simulink model "bh_model_crank_dynamics"  (R2022b)
settings: Solver=ode15s  StartTime=0.0  StopTime=45  RelTol=1e-4  AbsTol=1e-4  EnableMultiTasking=on
undefined symbols (not defined in the file): IC, params, sigbuilder_block, X, Y, Z
libraries: sm_lib x21, nesl_utility x19, simulink_extras x11, simulink x2
(part 2 of 2)

== system bh_model_crank_dynamics/BRAIN_model/INTEGRATE/Make_BUS/pm_pi ==
  rad_in : Inport
  Trigonometric Function : Trigonometry  Operator=atan2
  Trigonometric Function1 : Trigonometry
  Trigonometric Function2 : Trigonometry  Operator=cos
  rad_out : Outport
  wires:
  rad_in/1 -> Trigonometric Function2/1, Trigonometric Function1/1
  Trigonometric Function2/1 -> Trigonometric Function/2
  Trigonometric Function1/1 -> Trigonometric Function/1
  Trigonometric Function/1 -> rad_out/1

== system bh_model_crank_dynamics/BRAIN_model/INTEGRATE/Make_BUS/pm_pi1 ==
  rad_in : Inport
  Trigonometric Function : Trigonometry  Operator=atan2
  Trigonometric Function1 : Trigonometry
  Trigonometric Function2 : Trigonometry  Operator=cos
  rad_out : Outport
  wires:
  rad_in/1 -> Trigonometric Function2/1, Trigonometric Function1/1
  Trigonometric Function2/1 -> Trigonometric Function/2
  Trigonometric Function1/1 -> Trigonometric Function/1
  Trigonometric Function/1 -> rad_out/1

== matlab function bh_model_crank_dynamics/BRAIN_model/my_EOM1 ==
  data: F_P input; A output; I_A1 input; I_G2 input; L_1 input; L_2 input; b_A input; b_P input; g input; m_1 input; m_2 input; m_P input; tau_A input; theta input; theta_dot input; b output
function [A,b] = my_EOM(F_P,I_A1,I_G2,L_1,L_2,b_A,b_P,g,m_1,m_2,m_P,tau_A,theta,theta_dot)
%#codegen

%    This function was generated by the Symbolic Math Toolbox version 9.2.
%    27-Oct-2022 08:56:04

t2 = cos(theta);
t3 = sin(theta);
t4 = L_1.^2;
t5 = L_1.^3;
t6 = theta_dot.^2;
t10 = 1.0./L_2;
t7 = t2.^2;
t8 = t3.^2;
t9 = L_1.*t3;
t11 = t10.^2;
t12 = L_1.*t2.*t6;
t13 = t6.*t9;
t14 = t9./2.0;
t15 = t4.*t8.*t11;
t16 = -t15;
t17 = t15-1.0;
t18 = t16+1.0;
t19 = 1.0./t17;
t20 = sqrt(t18);
t23 = t3.*t5.*t6.*t7.*t11.*t19;
t21 = 1.0./t20;
t22 = (L_2.*t20)./2.0;
A = reshape([m_1.*t9.*(-1.0./2.0),(L_1.*m_1.*t2)./2.0,I_A1,-m_2.*(t9+(t2.*t3.*t4.*t10.*t21)./2.0),(L_1.*m_2.*t2)./2.0,-I_G2.*L_1.*t2.*t10.*t21,-m_P.*(t9+t2.*t3.*t4.*t10.*t21),0.0,-1.0,0.0,0.0,0.0,0.0,0.0,0.0,0.0,0.0,-1.0,0.0,0.0,0.0,0.0,0.0,0.0,1.0,0.0,-t9,-1.0,0.0,t14,0.0,0.0,0.0,1.0,L_1.*t2,0.0,-1.0,t22,0.0,0.0,0.0,0.0,0.0,1.0,0.0,t14,-1.0,0.0,0.0,0.0,0.0,0.0,1.0,t22,0.0,-1.0,0.0,0.0,0.0,0.0,0.0,0.0,0.0,-1.0],[8,8]);
if nargout > 1
    t24 = t13+t23;
    b = [(m_1.*t12)./2.0;-g.*m_1+(m_1.*t13)./2.0;tau_A-b_A.*theta_dot-(L_1.*g.*m_1.*t2)./2.0;m_2.*(t12-(t9.*t10.*t21.*t24)./2.0+(t4.*t6.*t7.*t10.*t21)./2.0);-g.*m_2+(m_2.*t13)./2.0;-I_G2.*t10.*t21.*t24;F_P+m_P.*(t12-t9.*t10.*t21.*t24+t4.*t6.*t7.*t10.*t21)+b_P.*(t9.*theta_dot+t2.*t3.*t4.*t10.*t21.*theta_dot);-g.*m_P];
end

== matlab function bh_model_crank_dynamics/SIMSCAPE_MODEL/make_R_BUS/Convert_BODY_fixed to WORLD ==
  data: xy_B_vec input size=2; xy_W_vec output size=[2,1]; gamma input size=1
function xy_W_vec = fcn(xy_B_vec, gamma)

    gRb      = [  cos(gamma),  -sin(gamma);
                  sin(gamma),   cos(gamma)   ];
      
    xy_W_vec = gRb * xy_B_vec(:);

end

== matlab function bh_model_crank_dynamics/BRAIN_model/INTEGRATE/CALC_P_pos_and_vel ==
  data: L_1 input; x_P output; L_2 input; theta input; theta_dot input; theta_ddot input; phi input; phi_dot input; v_P output; a_P output; phi_ddot input
function [x_P, v_P, a_P] = fcn(L_1, L_2, theta, theta_dot, theta_ddot, phi, phi_dot, phi_ddot)

    x_P =    L_1*cos(theta)  +  L_2*cos(phi);
    
    v_P =   -L_1*sin(theta)*theta_dot  - L_2*sin(phi)*phi_dot;  % need this for the damping Force
    
    a_P =   (-L_1*cos(theta)*theta_dot^2   + -L_1*sin(theta)*theta_ddot)   +   ...
            (-L_2*cos(phi)*phi_dot^2       + -L_2*sin(phi)*phi_ddot);

end

== matlab function bh_model_crank_dynamics/BRAIN_model/INTEGRATE/CALC_Phi_and_derivs ==
  data: theta input size=1; theta_dot input size=1; theta_ddot input size=1; L_1 input size=1; phi output double size=1; L_2 input size=1; phi_dot output double size=1; phi_ddot output double size=1
function [phi, phi_dot, phi_ddot] = fcn(theta,theta_dot,theta_ddot,L_1,L_2)

 phi      = asin(  (L_1/L_2) * sin(theta)  );

 phi_dot  = L_1*cos(theta)*theta_dot/(L_2*cos(phi));

 phi_ddot = (-L_1*sin(theta)*(theta_dot^2) + L_1*cos(theta)*theta_ddot + L_2*sin(phi)*(phi_dot^2))/(L_2*cos(phi));

end
